simulink model "IDENTIFICATION AND DISCRETE-TIME CONTROL OF A HEATING SYSTEM"  (R2016b)
settings: Solver=VariableStepAuto  StartTime=0.0  StopTime=400  RelTol=1e-3
values from neighbouring files (symbols this model uses):
  T = 1    [PID (Dynamic Method).m]
  x = [q0 q1 q2]    [PID (Dynamic Method).m]
settings Model: Creator=vovot  LastModifiedBy=vovot

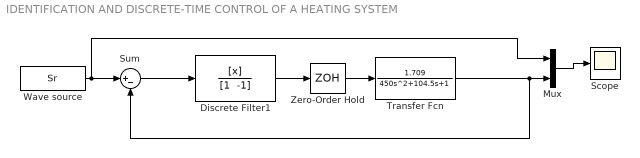
== system IDENTIFICATION AND DISCRETE-TIME CONTROL OF A HEATING SYSTEM ==
  Discrete Filter1 : DiscreteFilter  Numerator=[x]  Denominator="[1  -1]"  FilterStructure=Direct form I  SampleTime=T
  Mux : Mux  Inputs=2
  Scope : Scope
  Sum : Sum  Inputs=|+-
  Transfer Fcn : TransferFcn  Numerator=[1.709]  Denominator=[450 104.5 1]
  Wave source : FromWorkspace  VariableName=Sr  SampleTime=T
  Zero-Order Hold : ZeroOrderHold  SampleTime=T
  wires:
  Wave source/1 -> Mux/1, Sum/1
  Transfer Fcn/1 -> Mux/2, Sum/2
  Mux/1 -> Scope/1
  Sum/1 -> Discrete Filter1/1
  Discrete Filter1/1 -> Zero-Order Hold/1
  Zero-Order Hold/1 -> Transfer Fcn/1
